simulink model "model_1"  (R2013a)
settings: Solver=ode45  StartTime=0.0  StopTime=inf  RelTol=1e-3
libraries: simulink x3
settings Model: Creator=Claudiu  LastModifiedBy=Claudiu

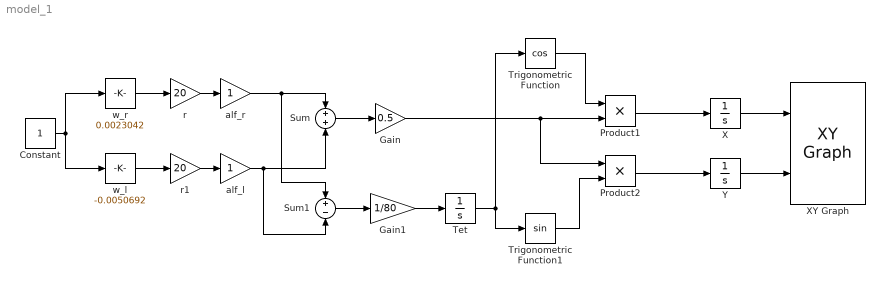
== system model_1 ==
  Constant : Constant
  Gain : Gain  Gain=0.5
  Gain1 : Gain  Gain=1/80
  Product1 : Product
  Product2 : Product
  Sum : Sum
  Sum1 : Sum  Inputs=+-
  Tet : Integrator
  Trigonometric Function : Trigonometry  Operator=cos
  Trigonometric Function1 : Trigonometry
  X : Integrator
  XY Graph : simulink/Sinks/XY Graph  xmin=-500  xmax=500  ymin=-500  ymax=500  st=-1
  Y : Integrator
  alf_l : Gain
  alf_r : Gain
  r : Gain  Gain=20
  r1 : Gain  Gain=20
  w_l : simulink/Math Operations/Slider Gain  low=-0.1  gain=-0.0050692  high=0.1
  w_r : simulink/Math Operations/Slider Gain  low=-0.1  gain=0.0023042  high=0.1
  wires:
  Y/1 -> XY Graph/2
  X/1 -> XY Graph/1
  Tet/1 -> Trigonometric Function/1, Trigonometric Function1/1
  Trigonometric Function/1 -> Product1/1
  Trigonometric Function1/1 -> Product2/2
  Sum/1 -> Gain/1
  Product1/1 -> X/1
  Product2/1 -> Y/1
  Constant/1 -> w_r/1, w_l/1
  w_r/1 -> r/1
  w_l/1 -> r1/1
  Sum1/1 -> Gain1/1
  Gain/1 -> Product2/1, Product1/2
  Gain1/1 -> Tet/1
  r/1 -> alf_r/1
  r1/1 -> alf_l/1
  alf_r/1 -> Sum1/1, Sum/1
  alf_l/1 -> Sum/2, Sum1/2
